simulink model "pendule_inv_capteur_etu"  (R2017a)
settings: Solver=VariableStepAuto  StartTime=0.0  StopTime=10.0  RelTol=1e-3
values from neighbouring files (symbols this model uses):
  K = [30 10]    [exemple_test_pendule_inv.m]    (also in exemple_test_pendule_inv_capteur.m = [10 1]; exemple_test_pendule_inv_echant.m)
  x0 = [pi/10 0]    [exemple_test_pendule_inv.m]    (also in exemple_test_pendule_inv_capteur.m = [pi/20 0]; exemple_test_pendule_inv_echant.m = [pi/20 0])
settings Model: Creator=aandre2  LastModifiedBy=aandre2

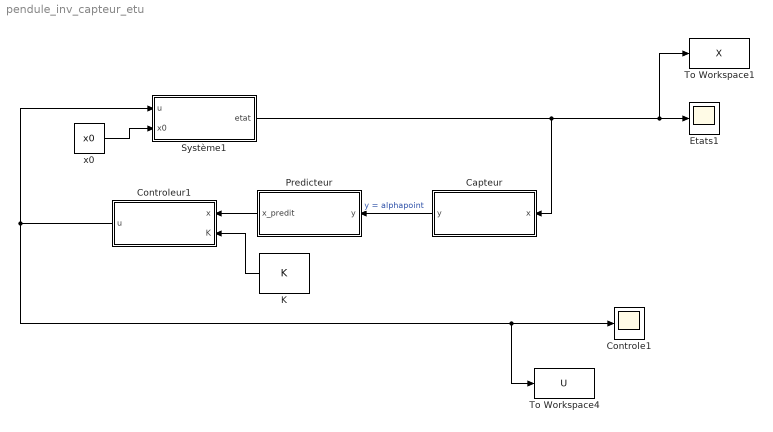
== system pendule_inv_capteur_etu ==
  Capteur : Subsystem
  Controle1 : Scope
  Controleur1 : Subsystem
  Etats1 : Scope
  K : Constant  Value=K
  Predicteur : Subsystem
  Système1 : Subsystem
  To Workspace1 : ToWorkspace  VariableName=X  SaveFormat=Timeseries  SampleTime=-1
  To Workspace4 : ToWorkspace  VariableName=U  SaveFormat=Timeseries  SampleTime=-1
  x0 : Constant  Value=x0
  wires:
  Controleur1/1(u) -> Système1/1(u), To Workspace4/1, Controle1/1
  Système1/1(etat) -> To Workspace1/1, Etats1/1, Capteur/1(x)
  Predicteur/1(x_predit) -> Controleur1/1(x)
  Capteur/1(y) -> Predicteur/1(y)  "y = alphapoint"
  x0/1 -> Système1/2(x0)
  K/1 -> Controleur1/2(K)

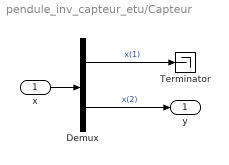
== system pendule_inv_capteur_etu/Capteur ==
  x : Inport
  Demux : Demux  Outputs=2
  Terminator : Terminator
  y : Outport
  wires:
  x/1 -> Demux/1
  Demux/2 -> y/1  "x(2)"
  Demux/1 -> Terminator/1  "x(1)"

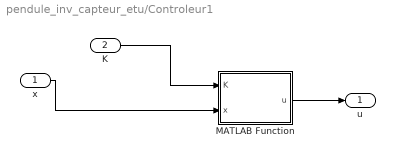
== system pendule_inv_capteur_etu/Controleur1 ==
  x : Inport
  K : Inport  Port=2
  MATLAB Function : MATLAB Function  TreatAsAtomicUnit=on
  u : Outport
  wires:
  MATLAB Function/1(u) -> u/1
  K/1 -> MATLAB Function/1(K)
  x/1 -> MATLAB Function/2(x)

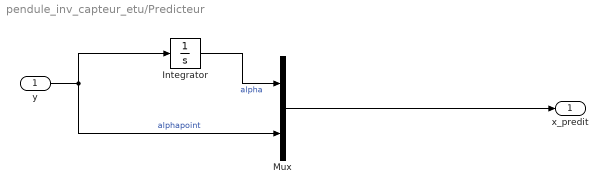
== system pendule_inv_capteur_etu/Predicteur ==
  y : Inport
  Integrator : Integrator
  Mux : Mux  Inputs=2
  x_predit : Outport
  wires:
  Integrator/1 -> Mux/1  "alpha"
  Mux/1 -> x_predit/1
  y/1 -> Integrator/1, Mux/2  "alphapoint"

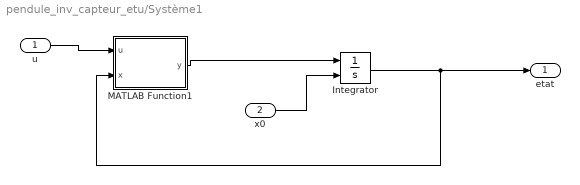
== system pendule_inv_capteur_etu/Système1 ==
  u : Inport
  x0 : Inport  Port=2
  Integrator : Integrator  InitialConditionSource=external
  MATLAB Function1 : MATLAB Function  TreatAsAtomicUnit=on
  etat : Outport  PortDimensions=2
  wires:
  MATLAB Function1/1(y) -> Integrator/1
  u/1 -> MATLAB Function1/1(u)
  Integrator/1 -> MATLAB Function1/2(x), etat/1
  x0/1 -> Integrator/2

== matlab function pendule_inv_capteur_etu/Controleur1/MATLAB Function ==
  data: K input; x input; u output
function u = fcn(K, x)
xe = [0 0];
ue= 0;
u = ue + K(1) * (x(1) - xe(1)) + K(2)*(x(2) -xe(2)) ;

== matlab function pendule_inv_capteur_etu/Système1/MATLAB Function1 ==
  data: u input; y output; x input
function y = fcn(u, x)
g = 9.81;
l = 10;
y = [0 0];
y(1) = x(2);
y(2) = g/l*sin(x(1))-cos(x(1))*u/l;
